simulink model "MoHinh_NhanDang_Cau2"  (R2018a)
settings: Solver=FixedStepAuto  StartTime=0  StopTime=100  FixedStep=0.01  RelTol=1e-3
values from neighbouring files (symbols this model uses):
  J1 = 0.03    [thongso_cau2.m]
  KB1 = 0.017    [thongso_cau2.m]
  KF1 = 0.25    [thongso_cau2.m]
  KM1 = 0.017    [thongso_cau2.m]
  L1 = 2.5    [thongso_cau2.m]
  R1 = 3    [thongso_cau2.m]
settings Model: OrderedModelArguments=off  Creator=20151  LastModifiedBy=20151
settings DataIOCC: ReturnWorkspaceOutputs=on
settings DebuggingCC: UnconnectedInputMsg=none  UnconnectedOutputMsg=none  UnconnectedLineMsg=none  SFMachineParentedDataDiag=error
settings SFSimCC: SimUseLocalCustomCode=on
settings RTWCC: RTWUseLocalCustomCode=on

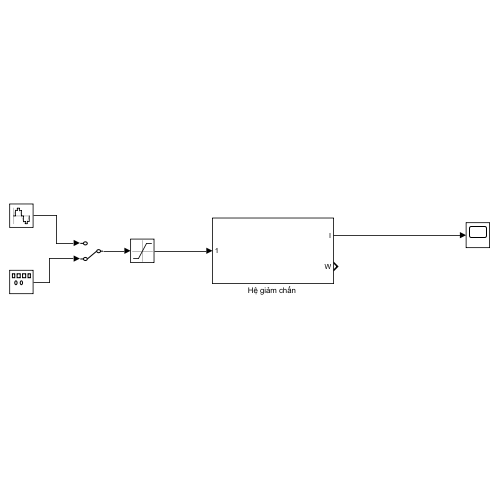
[thumbnail: Simulink's stored preview of the top-level diagram]
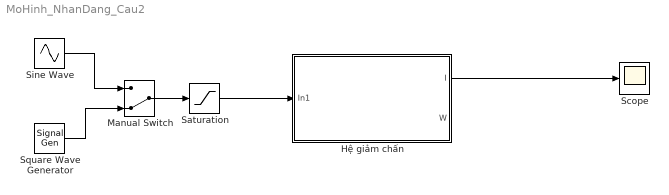
== system MoHinh_NhanDang_Cau2 ==
  "Hệ giảm chấn " : Subsystem
  Manual Switch : ManualSwitch  CurrentSetting=0
  Saturation : Saturate  UpperLimit=12  LowerLimit=-12
  Scope : Scope
  Sine Wave : Sin  SampleTime=0.01
  Square Wave Generator : SignalGenerator  WaveForm=random  Amplitude=20  Frequency=10  Units=rad/sec
  wires:
  Saturation/1 -> "Hệ giảm chấn "/1(In1)
  "Hệ giảm chấn "/1(I) -> Scope/1
  Square Wave Generator/1 -> Manual Switch/2
  Manual Switch/1 -> Saturation/1
  Sine Wave/1 -> Manual Switch/1

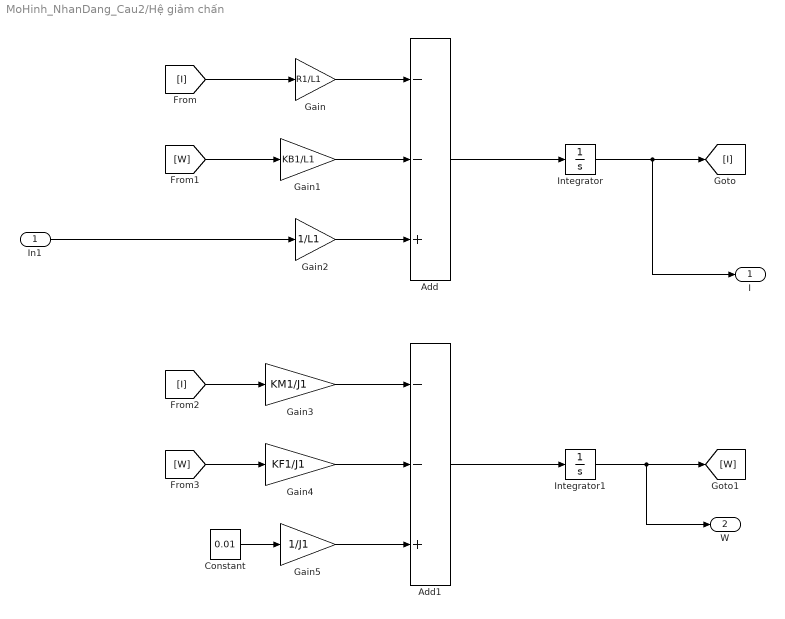
== system MoHinh_NhanDang_Cau2/Hệ giảm chấn  ==
  In1 : Inport
  Add : Sum  Inputs=--+
  Add1 : Sum  Inputs=--+
  Constant : Constant  Value=0.01
  Gain : Gain  Gain=R1/L1
  Gain1 : Gain  Gain=KB1/L1
  Gain2 : Gain  Gain=1/L1
  Gain3 : Gain  Gain=KM1/J1
  Gain4 : Gain  Gain=KF1/J1
  Gain5 : Gain  Gain=1/J1
  Integrator : Integrator
  Integrator1 : Integrator
  I : Outport
  W : Outport  Port=2
  wires:
  Gain/1 -> Add/1
  Gain1/1 -> Add/2
  Gain2/1 -> Add/3
  Gain3/1 -> Add1/1
  Gain4/1 -> Add1/2
  Gain5/1 -> Add1/3
  Add/1 -> Integrator/1
  Add1/1 -> Integrator1/1
  Integrator/1 -> I/1, [I]
  Integrator1/1 -> W/1, [W]
  [I] -> Gain/1
  [W] -> Gain1/1
  [W] -> Gain4/1
  [I] -> Gain3/1
  In1/1 -> Gain2/1
  Constant/1 -> Gain5/1
